simulink model "ITireAppMdl"  (R2017b)
settings: Solver=FixedStepDiscrete  StartTime=0.0  StopTime=10000  FixedStep=0.1  RelTol=1e-3
model workspace (MAT data in the model file):
  AilrflowValidFlag1 = [0.01235 0.03834 0.06233 0.08839 0.11261 0.13833 0.16348 0.18843 0.2134 0.23767 0.26241 0.28847 ... (108920 elements, 54460x2)]
  AilrflowValidFlag2 = [0.01258 0.03858 0.06256 0.08863 0.11285 0.13856 0.16371 0.18866 0.21363 0.2379 0.26264 0.2887 ... (108920 elements, 54460x2)]
  Airflow = [0.01258 0.03858 0.06256 0.08863 0.11285 0.13856 0.16371 0.18866 0.21363 0.2379 0.26264 0.2887 ... (108920 elements, 54460x2)]
  Frequency = [0.01235 0.03834 0.06233 0.08839 0.11261 0.13833 0.16348 0.18843 0.2134 0.23767 0.26241 0.28847 ... (108920 elements, 54460x2)]
  IntkAirHmdty = [0.07576 0.17591 0.27589 0.37591 0.47621 0.5753 0.67605 0.77531 0.87537 0.97532 1.07528 1.17533 ... (27230 elements, 13615x2)]
  IntkAirTemp = [0.07576 0.17591 0.27589 0.37591 0.47621 0.5753 0.67605 0.77531 0.87537 0.97532 1.07528 1.17533 ... (27230 elements, 13615x2)]
  IntkHmdtyTemp = [0.07576 0.17591 0.27589 0.37591 0.47621 0.5753 0.67605 0.77531 0.87537 0.97532 1.07528 1.17533 ... (27230 elements, 13615x2)]
  PriPresFilterValue = [0.01235 0.03834 0.06233 0.08839 0.11261 0.13833 0.16348 0.18843 0.2134 0.23767 0.26241 0.28847 ... (108920 elements, 54460x2)]
  PriPresRawValue = [0.01235 0.03834 0.06233 0.08839 0.11261 0.13833 0.16348 0.18843 0.2134 0.23767 0.26241 0.28847 ... (108920 elements, 54460x2)]
  SecPresFilterValue = [0.01258 0.03858 0.06256 0.08863 0.11285 0.13856 0.16371 0.18866 0.21363 0.2379 0.26264 0.2887 ... (108920 elements, 54460x2)]
  SecPresRawValue = [0.01258 0.03858 0.06256 0.08863 0.11285 0.13856 0.16371 0.18866 0.21363 0.2379 0.26264 0.2887 ... (108920 elements, 54460x2)]
  deltaPriPresFilterV = [0.01235 0.03834 0.06233 0.08839 0.11261 0.13833 0.16348 0.18843 0.2134 0.23767 0.26241 0.28847 ... (108920 elements, 54460x2)]
  deltaPriPresRawValu = [0.01235 0.03834 0.06233 0.08839 0.11261 0.13833 0.16348 0.18843 0.2134 0.23767 0.26241 0.28847 ... (108920 elements, 54460x2)]
  deltaSecPresFilterV = [0.01258 0.03858 0.06256 0.08863 0.11285 0.13856 0.16371 0.18866 0.21363 0.2379 0.26264 0.2887 ... (108920 elements, 54460x2)]
  deltaSecPresRawValu = [0.01258 0.03858 0.06256 0.08863 0.11285 0.13856 0.16371 0.18866 0.21363 0.2379 0.26264 0.2887 ... (108920 elements, 54460x2)]
values from neighbouring files (symbols this model uses):
  pTireHighPreDWLimit = 335.0    [ITiremyDictionary.sldd]
  pTireHighPreUpLimit = 350.0    [ITiremyDictionary.sldd]
  pTireLowPreDWLimit = 180.0    [ITiremyDictionary.sldd]
  pTireLowPreUpLimit = 195.0    [ITiremyDictionary.sldd]
(part 1 of 2)
settings Model: DataDictionary=ITiremyDictionary.sldd  Creator=xiangyinl  LastModifiedBy=VeHIL
settings DataIOCC: SaveOutput=off
settings OptimizationCC: BlockReduction=off  BooleanDataType=off  ConditionallyExecuteInputs=off  DefaultParameterBehavior=Inlined  UseDivisionForNetSlopeComputation=on  InlineInvariantSignals=on  OptimizeBlockIOStorage=off  BufferReuse=off  GlobalBufferReuse=off  ExpressionFolding=off  PassReuseOutputArgsAs=Individual arguments  LocalBlockOutputs=off  InitFltsAndDblsToZero=on  EfficientMapNaN2IntZero=off  LifeSpan=inf  BufferReusableBoundary=off  OptimizeDataStoreBuffers=off  BusAssignmentInplaceUpdate=off
settings DebuggingCC: SignalInfNanChecking=error  ReadBeforeWriteMsg=EnableAllAsError  WriteAfterWriteMsg=EnableAllAsError  WriteAfterReadMsg=EnableAllAsError  IntegerOverflowMsg=error  ParameterTunabilityLossMsg=error  UniqueDataStoreMsg=error  AssertControl=DisableAll  StrictBusMsg=ErrorOnBusTreatedAsVector  NonBusSignalsTreatedAsBus=error  SFInvalidInputDataAccessInChartInitDiag=error  SFTransitionOutsideNaturalParentDiag=error  SFUnreachableExecutionPathDiag=error  SFUndirectedBroadcastEventsDiag=error  SFOutputUsedAsStateInMooreChartDiag=none  IntegerSaturationMsg=error
settings HardwareCC: ProdBitPerPointer=32  ProdBitPerSizeT=32  ProdBitPerPtrDiffT=32  ProdLargestAtomicInteger=Integer  ProdWordSize=32  ProdHWDeviceType=STMicroelectronics->STM32 32-bit Cortex-M
settings ModelReferenceCC: ModelReferenceNumInstancesAllowed=Single
settings SFSimCC: MATLABDynamicMemAlloc=off
settings RTWCC: SystemTargetFile=ert.tlc  TemplateMakefile=ert_default_tmf  GenerateReport=on  Toolchain=Microsoft Visual C++ 2015 v14.0 | nmake (64-bit Windows)  IncludeHyperlinkInReport=on  LaunchReport=on  GenerateTraceInfo=on  GenerateTraceReport=on  GenerateTraceReportSl=on  GenerateTraceReportSf=on  GenerateTraceReportEml=on
settings CodeAppCC: ForceParamTrailComments=on  IgnoreCustomStorageClasses=off  OperatorAnnotations=on  SimulinkDataObjDesc=on  SFDataObjDesc=on  MATLABFcnDesc=on  InsertBlockDesc=on  StateflowObjectComments=on  MATLABSourceComments=on  EnableCustomComments=on  ReqsInCode=on
settings ERTTargetCC: TargetLangStandard=C99 (ISO)  GenerateSampleERTMain=on  CombineSignalStateStructs=on  SuppressErrorStatus=on  SupportNonFinite=off  ParenthesesLevel=Maximum  CastingMode=Standards  GenerateSharedConstants=off  ERTCustomFileTemplate=example_file_process.tlc  ERTFilePackagingFormat=Compact  ConvertIfToSwitch=off  EnableSignedLeftShifts=off  EnableSignedRightShifts=off

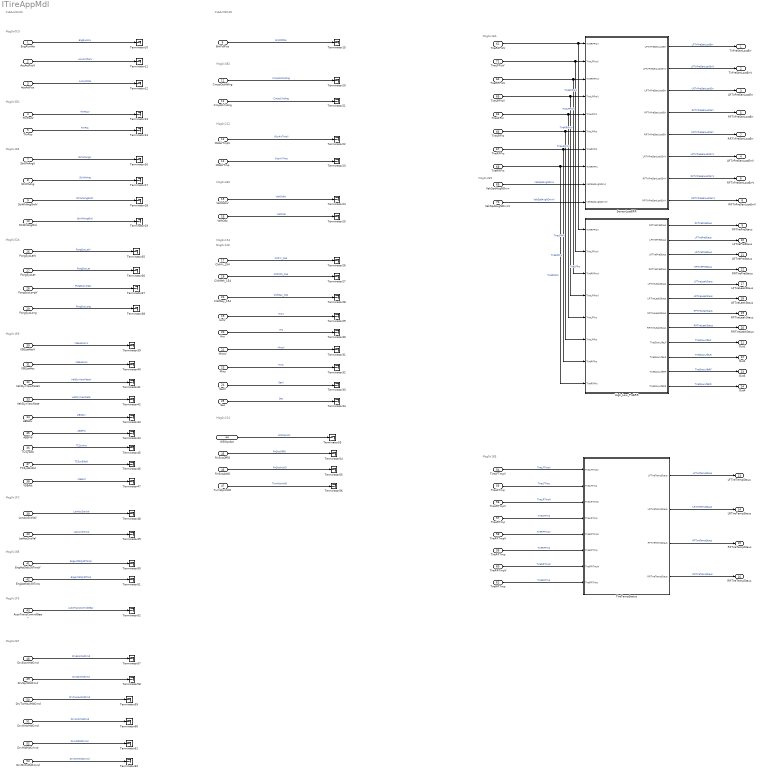
== system ITireAppMdl ==
  note: CLEA-HSCAN
  note: Msg0x3E9
  note: CLEA-MSCAN
  note: Msg0x1EA
  note: Msg0x0C9
  note: Msg0x3D1
  note: Msg0x128
  note: Msg0x1E5
  note: Msg0x382
  note: Msg0x212
  note: Msg0x360
  note: Msg0x154
  note: Msg0x32A
  note: Msg0x1E9
  note: Msg0x1FC
  note: Msg0x18E
  note: Msg0x1F5
  note: Msg0x214
  note: Msg0x287
  note: Msg0x1EE
  EngRunAtv : Inport  OutDataTypeStr=uint8
  AccActPosV : Inport  Port=2  OutDataTypeStr=uint8
  AccActPos : Inport  Port=3  OutDataTypeStr=uint8
  ThrPosV : Inport  Port=4  OutDataTypeStr=uint8
  ThrPos : Inport  Port=5  OutDataTypeStr=uint8
  BrkPdlPos : Inport  Port=6  OutDataTypeStr=uint8
  StrWhAngV : Inport  Port=7  OutDataTypeStr=uint8
  StrWhAng : Inport  Port=8  OutDataTypeStr=int16
  StrWhAngGrdV : Inport  Port=9  OutDataTypeStr=uint8
  StrWhAngGrd : Inport  Port=10  OutDataTypeStr=int16
  CmpsOctHding : Inport  Port=11  OutDataTypeStr=uint8
  CmpsCrhding : Inport  Port=12  OutDataTypeStr=uint16
  OtsAirTmpV : Inport  Port=13  OutDataTypeStr=uint8
  OtsAirTmp : Inport  Port=14  OutDataTypeStr=double
  VehOdoV : Inport  Port=15  OutDataTypeStr=uint8
  VehOdo : Inport  Port=16  OutDataTypeStr=uint32
  CldrYr_154 : Inport  Port=17  OutDataTypeStr=uint16
  CldrMth_154 : Inport  Port=18  OutDataTypeStr=uint8
  HrsV : Inport  Port=19  OutDataTypeStr=uint8
  Hrs : Inport  Port=20  OutDataTypeStr=uint8
  MinsV : Inport  Port=21  OutDataTypeStr=uint8
  CldrDay_154 : Inport  Port=22  OutDataTypeStr=uint8
  Mins : Inport  Port=23  OutDataTypeStr=uint8
  SecV : Inport  Port=24  OutDataTypeStr=uint8
  Sec : Inport  Port=25  OutDataTypeStr=uint8
  PsngSysLatV : Inport  Port=26  OutDataTypeStr=uint8
  PsngSysLat : Inport  Port=27  OutDataTypeStr=int32
  PsngSysLongV : Inport  Port=28  OutDataTypeStr=uint8
  PsngSysLong : Inport  Port=29  OutDataTypeStr=int32
  VSELatAccV : Inport  Port=30  OutDataTypeStr=uint8
  VSELatAcc : Inport  Port=31  OutDataTypeStr=double
  VehDynYawRateV : Inport  Port=32  OutDataTypeStr=uint8
  VehDynYawRate : Inport  Port=33  OutDataTypeStr=double
  ABSAtv : Inport  Port=34  OutDataTypeStr=uint8
  ABSFld : Inport  Port=35  OutDataTypeStr=uint8
  TCSysAtv : Inport  Port=36  OutDataTypeStr=uint8
  TCSysEnbld : Inport  Port=37  OutDataTypeStr=uint8
  VSEAct : Inport  Port=38  OutDataTypeStr=uint8
  LonAccSnsVal : Inport  Port=39  OutDataTypeStr=double
  LatAccSnsVal : Inport  Port=40  OutDataTypeStr=double
  EngActStdyStTorqV : Inport  Port=41  OutDataTypeStr=uint8
  EngActStdyStTorq : Inport  Port=42  OutDataTypeStr=double
  AutoTransComndGear : Inport  Port=43  OutDataTypeStr=uint8
  WSWprAct : Inport  Port=44  OutDataTypeStr=uint8
  RnSnsOffIO : Inport  Port=45
  RnSnsActIO : Inport  Port=46
  TurnWprIntIO : Inport  Port=47
  DrvEconMdCmd : Inport  Port=48  OutDataTypeStr=uint8
  DrvSprtMdCmd : Inport  Port=49  OutDataTypeStr=uint8
  DrvTwHaulMdCmd : Inport  Port=50  OutDataTypeStr=uint8
  DrvWntrMdCmd : Inport  Port=51  OutDataTypeStr=uint8
  DrvHldMdCmnd : Inport  Port=52  OutDataTypeStr=uint8
  DrvMntnMdCmnd : Inport  Port=53  OutDataTypeStr=uint8
  TireLFTmpV : Inport  Port=54  OutDataTypeStr=uint8
  TireLFTmp : Inport  Port=55  OutDataTypeStr=int16
  TireLRTmpV : Inport  Port=56  OutDataTypeStr=uint8
  TireLRTmp : Inport  Port=57  OutDataTypeStr=int16
  TireRFTmpV : Inport  Port=58  OutDataTypeStr=uint8
  TireRFTmp : Inport  Port=59  OutDataTypeStr=int16
  TireRRTmpV : Inport  Port=60  OutDataTypeStr=uint8
  TireRRTmp : Inport  Port=61  OutDataTypeStr=int16
  TireRFPrsV : Inport  Port=62
  TireLFPrs : Inport  Port=63
  TireRRPrsV : Inport  Port=64
  TireLRPrsV : Inport  Port=65
  TireLRPrs : Inport  Port=66
  TireRFPrs : Inport  Port=67
  TireRRPrs : Inport  Port=68
  VehSpdAvgNDrvn : Inport  Port=69
  VehSpdAvgNDrvnV : Inport  Port=70  OutDataTypeStr=uint8
  TireLFPrsV : Inport  Port=71
  High_Low_PrsERR : Stateflow chart  TreatAsAtomicUnit=on
  SensorLostERR : Stateflow chart  TreatAsAtomicUnit=on
  Terminator{10..62} (53 alike) : Terminator
  TireTempStatus : Stateflow chart  TreatAsAtomicUnit=on
  TirPreSenLostErr : Outport  OutDataTypeStr=uint8
  TirPreSenLostErrV : Outport  Port=2  OutDataTypeStr=uint8
  LRTirPreSenLostErr : Outport  Port=3  OutDataTypeStr=uint8
  LRTirPreSenLostErrV : Outport  Port=4  OutDataTypeStr=uint8
  RFTirPreSenLostErr : Outport  Port=5  OutDataTypeStr=uint8
  RFTirPreSenLostErrV : Outport  Port=6  OutDataTypeStr=uint8
  RRTirPreSenLostErr : Outport  Port=7  OutDataTypeStr=uint8
  RRTirPreSenLostErrV : Outport  Port=8  OutDataTypeStr=uint8
  RFTirePreStaus : Outport  Port=9  OutDataTypeStr=uint8
  LFTirePreStaus : Outport  Port=10
  LRTirePreStaus : Outport  Port=11
  RRTirePreStaus : Outport  Port=12
  LFTireTempStaus : Outport  Port=13
  LRTireTempStaus : Outport  Port=14
  RFTireTempStaus : Outport  Port=15
  RRTireTempStaus : Outport  Port=16
  LFTireLeakStaus : Outport  Port=17  OutDataTypeStr=uint8
  LRTireLeakStaus : Outport  Port=18  OutDataTypeStr=uint8
  RFTireLeakStaus : Outport  Port=19  OutDataTypeStr=uint8
  RRTireLeakStaus : Outport  Port=20  OutDataTypeStr=uint8
  Out1 : Outport  Port=21
  Out2 : Outport  Port=22
  Out3 : Outport  Port=23
  Out4 : Outport  Port=24
  wires:
  VehSpdAvgNDrvnV/1 -> SensorLostERR/10(VehSpdAvgNDrvnV)  "VehSpdAvgNDrvnV"
  VehSpdAvgNDrvn/1 -> SensorLostERR/9(VehSpdAvgNDrvn)  "VehSpdAvgNDrvn"
  TireRFPrsV/1 -> High_Low_PrsERR/1(TireRFPrsV), SensorLostERR/1(TireRFPrsV)  "TireRFPrsV"
  TireLFPrsV/1 -> High_Low_PrsERR/2(TireLFPrsV), SensorLostERR/2(TireLFPrsV)  "TireLFPrsV"
  TireRRPrsV/1 -> High_Low_PrsERR/3(TireRRPrsV), SensorLostERR/3(TireRRPrsV)  "TireRRPrsV"
  TireLRPrsV/1 -> High_Low_PrsERR/4(TireLRPrsV), SensorLostERR/4(TireLRPrsV)  "TireLRPrsV"
  TireLFPrs/1 -> High_Low_PrsERR/5(TireLFPrs), SensorLostERR/5(TireLFPrs)  "TireLFPrs"
  TireLRPrs/1 -> High_Low_PrsERR/6(TireLRPrs), SensorLostERR/6(TireLRPrs)  "TireLRPrs"
  TireRFPrs/1 -> High_Low_PrsERR/7(TireRFPrs), SensorLostERR/7(TireRFPrs)  "TireRFPrs"
  TireRRPrs/1 -> High_Low_PrsERR/8(TireRRPrs), SensorLostERR/8(TireRRPrs)  "TireRRPrs"
  EngRunAtv/1 -> Terminator10/1  "EngRunAtv"
  AccActPosV/1 -> Terminator11/1  "AccActPosV"
  AccActPos/1 -> Terminator12/1  "AccActPos"
  ThrPosV/1 -> Terminator13/1  "ThrPosV"
  ThrPos/1 -> Terminator14/1  "ThrPos"
  BrkPdlPos/1 -> Terminator15/1  "BrkPdlPos"
  StrWhAngV/1 -> Terminator16/1  "StrWhAngV"
  StrWhAng/1 -> Terminator17/1  "StrWhAng"
  StrWhAngGrdV/1 -> Terminator18/1  "StrWhAngGrdV"
  StrWhAngGrd/1 -> Terminator19/1  "StrWhAngGrd"
  CmpsOctHding/1 -> Terminator20/1  "CmpsOctHding"
  CmpsCrhding/1 -> Terminator21/1  "CmpsCrhding"
  OtsAirTmpV/1 -> Terminator22/1  "OtsAirTmpV"
  OtsAirTmp/1 -> Terminator23/1  "OtsAirTmp"
  VehOdoV/1 -> Terminator24/1  "VehOdoV"
  VehOdo/1 -> Terminator25/1  "VehOdo"
  CldrYr_154/1 -> Terminator26/1  "CldrYr_154"
  CldrMth_154/1 -> Terminator27/1  "CldrMth_154"
  HrsV/1 -> Terminator29/1  "HrsV"
  Hrs/1 -> Terminator30/1  "Hrs"
  MinsV/1 -> Terminator31/1  "MinsV"
  CldrDay_154/1 -> Terminator28/1  "CldrDay_154"
  Mins/1 -> Terminator32/1  "Mins"
  SecV/1 -> Terminator33/1  "SecV"
  Sec/1 -> Terminator34/1  "Sec"
  PsngSysLatV/1 -> Terminator35/1  "PsngSysLatV"
  PsngSysLat/1 -> Terminator36/1  "PsngSysLat"
  PsngSysLongV/1 -> Terminator37/1  "PsngSysLongV"
  PsngSysLong/1 -> Terminator38/1  "PsngSysLong"
  VSELatAccV/1 -> Terminator39/1  "VSELatAccV"
  VSELatAcc/1 -> Terminator40/1  "VSELatAcc"
  VehDynYawRateV/1 -> Terminator41/1  "VehDynYawRateV"
  VehDynYawRate/1 -> Terminator42/1  "VehDynYawRate"
  ABSAtv/1 -> Terminator43/1  "ABSAtv"
  ABSFld/1 -> Terminator44/1  "ABSFld"
  TCSysAtv/1 -> Terminator45/1  "TCSysAtv"
  TCSysEnbld/1 -> Terminator46/1  "TCSysEnbld"
  VSEAct/1 -> Terminator47/1  "VSEAct"
  LonAccSnsVal/1 -> Terminator48/1  "LonAccSnsVal"
  LatAccSnsVal/1 -> Terminator49/1  "LatAccSnsVal"
  EngActStdyStTorqV/1 -> Terminator50/1  "EngActStdyStTorqV"
  EngActStdyStTorq/1 -> Terminator51/1  "EngActStdyStTorq"
  AutoTransComndGear/1 -> Terminator52/1  "AutoTransComndGear"
  WSWprAct/1 -> Terminator53/1  "WSWprAct"
  RnSnsOffIO/1 -> Terminator54/1  "RnSnsOffIO"
  RnSnsActIO/1 -> Terminator55/1  "RnSnsActIO"
  TurnWprIntIO/1 -> Terminator56/1  "TurnWprIntIO"
  DrvEconMdCmd/1 -> Terminator57/1  "DrvEconMdCmd"
  DrvSprtMdCmd/1 -> Terminator58/1  "DrvSprtMdCmd"
  DrvTwHaulMdCmd/1 -> Terminator59/1  "DrvTwHaulMdCmd"
  DrvWntrMdCmd/1 -> Terminator60/1  "DrvWntrMdCmd"
  DrvHldMdCmnd/1 -> Terminator61/1  "DrvHldMdCmnd"
  DrvMntnMdCmnd/1 -> Terminator62/1  "DrvMntnMdCmnd"
  TireLFTmpV/1 -> TireTempStatus/1(TireLFTmpV)  "TireLFTmpV"
  TireLFTmp/1 -> TireTempStatus/2(TireLFTmp)  "TireLFTmp"
  TireLRTmpV/1 -> TireTempStatus/3(TireLRTmpV)  "TireLRTmpV"
  TireLRTmp/1 -> TireTempStatus/4(TireLRTmp)  "TireLRTmp"
  TireRFTmpV/1 -> TireTempStatus/5(TireRFTmpV)  "TireRFTmpV"
  TireRFTmp/1 -> TireTempStatus/6(TireRFTmp)  "TireRFTmp"
  TireRRTmpV/1 -> TireTempStatus/7(TireRRTmpV)  "TireRRTmpV"
  TireRRTmp/1 -> TireTempStatus/8(TireRRTmp)  "TireRRTmp"
  SensorLostERR/1(LFTirPreSenLostErr) -> TirPreSenLostErr/1  "LFTirPreSenLostErr"
  SensorLostERR/2(LFTirPreSenLostErrV) -> TirPreSenLostErrV/1  "LFTirPreSenLostErrV"
  SensorLostERR/3(LRTirPreSenLostErr) -> LRTirPreSenLostErr/1  "LRTirPreSenLostErr"
  SensorLostERR/4(RFTirPreSenLostErr) -> RFTirPreSenLostErr/1  "RFTirPreSenLostErr"
  SensorLostERR/6(LRTirPreSenLostErrV) -> LRTirPreSenLostErrV/1  "LRTirPreSenLostErrV"
  SensorLostERR/5(RRTirPreSenLostErr) -> RRTirPreSenLostErr/1  "RRTirPreSenLostErr"
  SensorLostERR/7(RFTirPreSenLostErrV) -> RFTirPreSenLostErrV/1  "RFTirPreSenLostErrV"
  SensorLostERR/8(RRTirPreSenLostErrV) -> RRTirPreSenLostErrV/1  "RRTirPreSenLostErrV"
  High_Low_PrsERR/1(RFTirePreStaus) -> RFTirePreStaus/1  "RFTirePreStaus"
  High_Low_PrsERR/2(LFTirePreStaus) -> LFTirePreStaus/1  "LFTirePreStaus"
  High_Low_PrsERR/3(LRTirePreStaus) -> LRTirePreStaus/1  "LRTirePreStaus"
  High_Low_PrsERR/4(RRTirePreStaus) -> RRTirePreStaus/1  "RRTirePreStaus"
  TireTempStatus/1(LFTireTempStaus) -> LFTireTempStaus/1  "LFTireTempStaus"
  TireTempStatus/2(LRTireTempStaus) -> LRTireTempStaus/1  "LRTireTempStaus"
  TireTempStatus/3(RFTireTempStaus) -> RFTireTempStaus/1  "RFTireTempStaus"
  TireTempStatus/4(RRTireTempStaus) -> RRTireTempStaus/1  "RRTireTempStaus"
  High_Low_PrsERR/5(LFTireLeakStaus) -> LFTireLeakStaus/1  "LFTireLeakStaus"
  High_Low_PrsERR/6(LRTireLeakStaus) -> LRTireLeakStaus/1  "LRTireLeakStaus"
  High_Low_PrsERR/7(RFTireLeakStaus) -> RFTireLeakStaus/1  "RFTireLeakStaus"
  High_Low_PrsERR/8(RRTireLeakStaus) -> RRTireLeakStaus/1  "RRTireLeakStaus"
  High_Low_PrsERR/9(TireSlowLifeLF) -> Out1/1  "TireSlowLifeLF"
  High_Low_PrsERR/10(TireSlowLifeLR) -> Out2/1  "TireSlowLifeLR"
  High_Low_PrsERR/11(TireSlowLifeRF) -> Out3/1  "TireSlowLifeRF"
  High_Low_PrsERR/12(TireSlowLifeRR) -> Out4/1  "TireSlowLifeRR"
